simulink model "robot_model"  (R2021b)
settings: Solver=VariableStepAuto  StartTime=0.0  StopTime=10.0  RelTol=1e-3
libraries: robotmaniplib x1
settings Model: Creator=jcron  LastModifiedBy=jcron

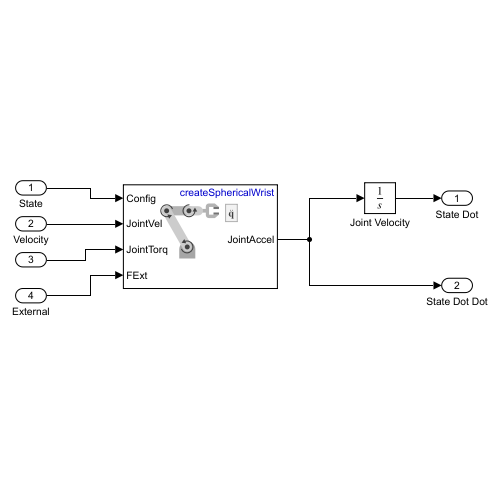
[thumbnail: Simulink's stored preview of the top-level diagram]
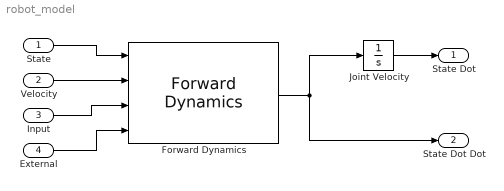
== system robot_model ==
  State : Inport
  Velocity : Inport  Port=2
  Input : Inport  Port=3
  External : Inport  Port=4
  Forward Dynamics : robotmaniplib/Forward Dynamics  RigidBodyTree=createSphericalWrist  SimulateUsing=Interpreted execution
  Joint Velocity : Integrator
  State Dot : Outport  PortDimensions=DOF
  State Dot Dot : Outport  Port=2  PortDimensions=DOF
  wires:
  State/1 -> Forward Dynamics/1
  Velocity/1 -> Forward Dynamics/2
  Input/1 -> Forward Dynamics/3
  Joint Velocity/1 -> State Dot/1
  Forward Dynamics/1 -> State Dot Dot/1, Joint Velocity/1
  External/1 -> Forward Dynamics/4
